simulink model "softarm_tendon_acceleration_demo"  (R2025a)
settings: Solver=ode15s  StartTime=0.0  StopTime=0.5  RelTol=1e-3
PreLoadFcn:
  | softarm_root=fileparts(get_param(bdroot,'FileName'));addpath(softarm_root);addpath(fullfile(softarm_root,'matlab'));
InitFcn:
  | softarm_root=fileparts(get_param(bdroot,'FileName'));addpath(fullfile(softarm_root,'matlab'));softarm_plant_block=string(bdroot)+"/Plant";softarm.applyPlantMask(softarm_plant_block,'strict');
undefined symbols (not defined in the file or in its folder): softarm_narm, softarm_nq, softarm_nu, softarm_x0
settings Model: Creator=rlwan  LastModifiedBy=rlwan

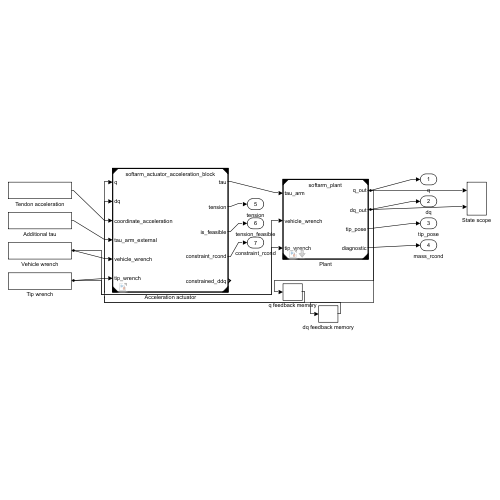
[thumbnail: Simulink's stored preview of the top-level diagram]
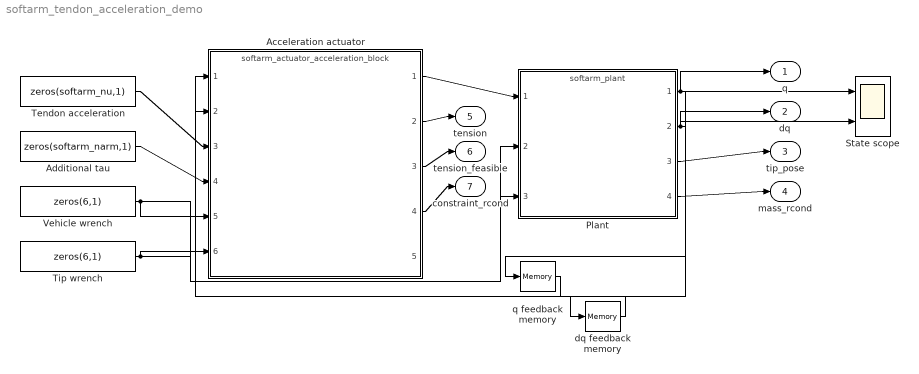
== system softarm_tendon_acceleration_demo ==
  Acceleration actuator : ModelReference  ModelNameDialog=softarm_actuator_acceleration_block  ModelReferenceVersion=1.1
  Additional tau : Constant  Value=zeros(softarm_narm,1)
  Plant : ModelReference  ModelNameDialog=softarm_plant  ParameterArgumentNames=Bundle  ParameterArgumentValues=Bundle  UsingDefaultArgumentValue=0  ModelReferenceVersion=1.1  Bundle='examples/generated/pcc_three_tendon_extensible_n2'
  State scope : Scope  NumInputPorts=2
  Tendon acceleration : Constant  Value=zeros(softarm_nu,1)
  Tip wrench : Constant  Value=zeros(6,1)
  Vehicle wrench : Constant  Value=zeros(6,1)
  dq feedback memory : Memory  InitialCondition=zeros(softarm_nq,1)
  q feedback memory : Memory  InitialCondition=softarm_x0(1:softarm_nq)
  q : Outport
  dq : Outport  Port=2
  tip_pose : Outport  Port=3
  mass_rcond : Outport  Port=4
  tension : Outport  Port=5
  tension_feasible : Outport  Port=6
  constraint_rcond : Outport  Port=7
  wires:
  Plant/1 -> q feedback memory/1, q/1, State scope/1
  q feedback memory/1 -> Acceleration actuator/1
  Plant/2 -> dq feedback memory/1, dq/1, State scope/2
  dq feedback memory/1 -> Acceleration actuator/2
  Tendon acceleration/1 -> Acceleration actuator/3
  Additional tau/1 -> Acceleration actuator/4
  Vehicle wrench/1 -> Acceleration actuator/5, Plant/2
  Tip wrench/1 -> Acceleration actuator/6, Plant/3
  Acceleration actuator/1 -> Plant/1
  Acceleration actuator/2 -> tension/1
  Acceleration actuator/3 -> tension_feasible/1
  Acceleration actuator/4 -> constraint_rcond/1
  Plant/3 -> tip_pose/1
  Plant/4 -> mass_rcond/1
